simulink model "mpc_period_exp_simulink"  (R2015a)
settings: Solver=ode45  SolverMode=SingleTasking  StartTime=0.0  StopTime=simu.simulation_time  RelTol=1e-3
values from neighbouring files (symbols this model uses):
  plant = tf([2 3],[a 5 1])    [mpc_period_abitary_input.m]    (also in mpc_period_exp.m = tf([3], [tau 1]); mpc_period_with_abitary_reference.m = tf([10],[tau 1]))
undefined symbols (not defined in the file or in its folder): simu
libraries: simulink x1, mpclib x1
settings Model: CovSFcnEnable=off  ExtModeTrigMode=oneshot  ExtModeArmWhenConnect=off  Creator=The MathWorks Inc.  LastModifiedBy=Xiaotian
settings DataIOCC: LimitDataPoints=off  SaveOutput=off  SignalLogging=off  DSMLogging=off  SaveTime=off  SignalLoggingName=sigsOut
settings OptimizationCC: BooleanDataType=off  ExpressionDepthLimit=2147483647  InitFltsAndDblsToZero=on
settings DebuggingCC: SaveWithParameterizedLinksMsg=none  UnderspecifiedInitializationDetection=Classic  MergeDetectMultiDrivingBlocksExec=none  SignalResolutionControl=TryResolveAllWithWarning  MultiTaskDSMMsg=warning  MultiTaskCondExecSysMsg=none  IntegerOverflowMsg=none  FcnCallInpInsideContextMsg=UseLocalSettings  StateNameClashWarn=warning  IntegerSaturationMsg=none
settings HardwareCC: TargetUnknown=on
settings GRTTargetCC: TargetFcnLib=ansi_tfl_tmw.mat  CombineOutputUpdateFcns=off  GRTInterface=on

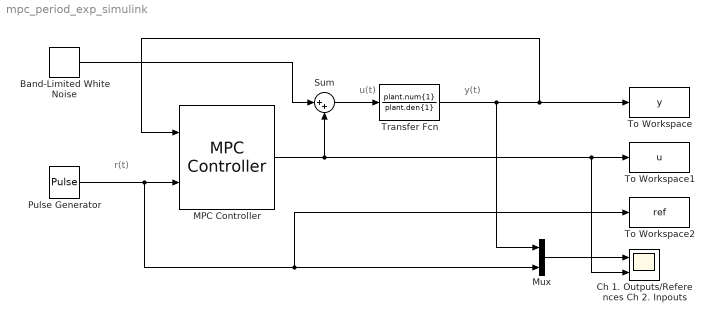
== system mpc_period_exp_simulink ==
  note: u(t)
  note: y(t)
  note: r(t)
  Band-Limited White Noise : simulink/Sources/Band-Limited White Noise  Cov=[simu.noise_level]  Ts=10  seed=[23341]
  Ch 1. Outputs/References Ch 2. Inpouts : Scope  NumInputPorts=2
      settings: TimeRange=10  YMin=0~-5  YMax=1.5~5  DataFormat=Structure  SampleInput=on  SampleTime=0.01
  MPC Controller : mpclib/MPC Controller  mpcobj=mpcobj  x0=[]  is_multiple=0  enable_value=0  n_mv=1  n_mo=1  n_md=0  n_ts=3.6  is_designfromscratch=0  return_u0=off  ref_from_ws=off  ref_signal_name=[]  ref_preview=on  md_from_ws=off  md_signal_name=[]  md_preview=on  from_project=off  project_file=MPCtask.mat  md_inport=off  mv_inport=off  cost_outport=off  return_sequence=off  return_qpstatus=off  return_state=off  state_inport=off  lims_inport=off  ywt_inport=off  uwt_inport=off  duwt_inport=off  rhoeps_inport=off  uref_inport=off  BlockDataType=double  SampleTimeInherited=off  switch_inport=off
  Mux : Mux  Inputs=2
  Pulse Generator : DiscretePulseGenerator  PulseType=Time based  Period=50  PulseWidth=50  PhaseDelay=1  VectorParams1D=off
  Sum : Sum  Inputs=|++
  To Workspace : ToWorkspace  VariableName=y  SaveFormat=Timeseries  SampleTime=simu.samlping_time
      settings: MaxDataPoints=Inf
  To Workspace1 : ToWorkspace  VariableName=u  SaveFormat=Timeseries  SampleTime=simu.samlping_time
      settings: MaxDataPoints=Inf
  To Workspace2 : ToWorkspace  VariableName=ref  SaveFormat=Timeseries  SampleTime=simu.samlping_time
      settings: MaxDataPoints=Inf
  Transfer Fcn : TransferFcn  Numerator=plant.num{1}  Denominator=plant.den{1}
  wires:
  MPC Controller/1 -> Sum/2, Ch 1. Outputs/References Ch 2. Inpouts/2, To Workspace1/1
  Transfer Fcn/1 -> To Workspace/1, MPC Controller/1, Mux/1
  Mux/1 -> Ch 1. Outputs/References Ch 2. Inpouts/1
  Pulse Generator/1 -> To Workspace2/1, Mux/2, MPC Controller/2
  Band-Limited White Noise/1 -> Sum/1
  Sum/1 -> Transfer Fcn/1
